simulink model "q8"  (Simulink 8.1)
settings: Solver=ode45  StartTime=0.0  StopTime=10.0  RelTol=1e-3
values from neighbouring files (symbols this model uses):
  Kq8 = 0.7*N^(-a)    (= 0.7)    [task2.m]
settings Model: Creator=Nelson  LastModifiedBy=Nelson
settings DataIOCC: SignalLoggingSaveFormat=Dataset
settings OptimizationCC: ExpressionDepthLimit=128
settings DebuggingCC: FcnCallInpInsideContextMsg=EnableAllAsError
settings GRTTargetCC: CombineOutputUpdateFcns=on  GRTInterface=off

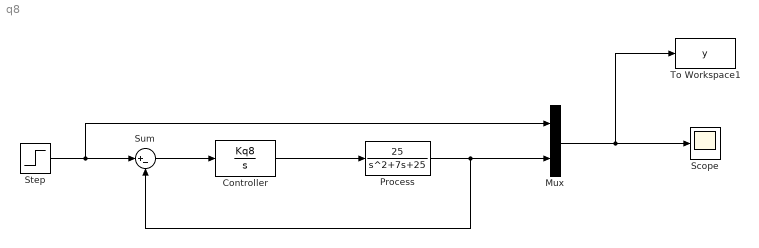
== system q8 ==
  Controller : TransferFcn  Numerator=Kq8  Denominator=[1 0]
  Mux : Mux  Inputs=2
  Process : TransferFcn  Numerator=[25]  Denominator=[1 7 25]
  Scope : Scope
  Step : Step  Time=0  SampleTime=0
  Sum : Sum  Inputs=|+-
  To Workspace1 : ToWorkspace  VariableName=y  SampleTime=-1
  wires:
  Process/1 -> Sum/2, Mux/2
  Controller/1 -> Process/1
  Sum/1 -> Controller/1
  Step/1 -> Sum/1, Mux/1
  Mux/1 -> Scope/1, To Workspace1/1
